simulink model "capteur"  (R2020b)
settings: Solver=VariableStepAuto  StartTime=0.0  StopTime=5  RelTol=1e-3
settings Model: Creator=simon  LastModifiedBy=simon

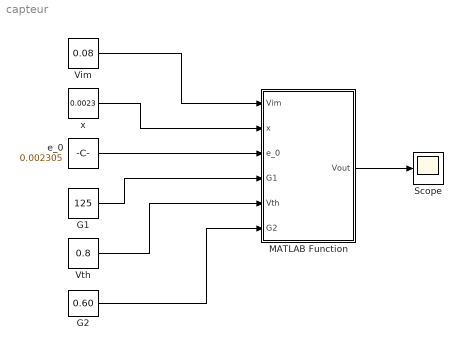
== system capteur ==
  G1 : Constant  Value=125
  G2 : Constant  Value=0.60
  MATLAB Function : MATLAB Function  TreatAsAtomicUnit=on
  Scope : Scope
  Vim : Constant  Value=0.08
  Vth : Constant  Value=0.8
  e_0 : Constant  Value=0.002305
  x : Constant  Value=0.0023
  wires:
  e_0/1 -> MATLAB Function/3(e_0)
  x/1 -> MATLAB Function/2(x)
  Vim/1 -> MATLAB Function/1(Vim)
  G1/1 -> MATLAB Function/4(G1)
  Vth/1 -> MATLAB Function/5(Vth)
  G2/1 -> MATLAB Function/6(G2)
  MATLAB Function/1(Vout) -> Scope/1

== matlab function capteur/MATLAB Function ==
  data: Vim input; Vout output; x input; e_0 input; G1 input; Vth input; G2 input
function Vout = fcn(Vim,x,e_0,G1,Vth,G2)

Vout = ((Vim/2)*(1+x/e_0)*G1 - Vth)*G2;
